simulink model "drive_force_start"  (R2018a)
settings: Solver=ode45  StartTime=0.0  StopTime=15  RelTol=1e-3  EnableMultiTasking=on
PreLoadFcn:
  | load gear_data;
  | FDR = 3.23;
  | AvgEngTorque = 222;
  | Loss = 0.8;
  | r_tire = 1.030;
settings Model: Creator=jrivitus  LastModifiedBy=bneiswan
settings DataIOCC: ExternalInput=[t, gear]  LimitDataPoints=on  LoadExternalInput=on  SaveFormat=Array
settings OptimizationCC: ExpressionDepthLimit=2147483647  LifeSpan=inf
settings DebuggingCC: UnderspecifiedInitializationDetection=Classic  MergeDetectMultiDrivingBlocksExec=none  ParameterPrecisionLossMsg=none  FcnCallInpInsideContextMsg=warning  AllowSymbolicDim=off  StateNameClashWarn=warning  SFUnexpectedBacktrackingDiag=warning  SFNoUnconditionalDefaultTransitionDiag=warning  SFExecutionAtInitializationDiag=none
settings HardwareCC: ProdBitPerPointer=32  ProdBitPerSizeT=32  ProdBitPerPtrDiffT=32  ProdLargestAtomicFloat=None  ProdIntDivRoundTo=Undefined  ProdEndianess=Unspecified  ProdWordSize=32  ProdHWDeviceType=32-bit Generic
settings ModelReferenceCC: PropagateSignalLabelsOutOfModel=off
settings CodeAppCC: StateflowObjectComments=on
settings GRTTargetCC: TargetLangStandard=C89/C90 (ANSI)  GeneratePreprocessorConditionals=Disable all  CombineOutputUpdateFcns=off  GRTInterface=on
settings ConfigComp: CovMetricSettings=dw  CovHtmlReporting=on  CovSaveCumulativeToWorkspaceVar=on  CovSaveSingleToWorkspaceVar=on  CovExternalEMLEnable=off  CovSFcnEnable=off

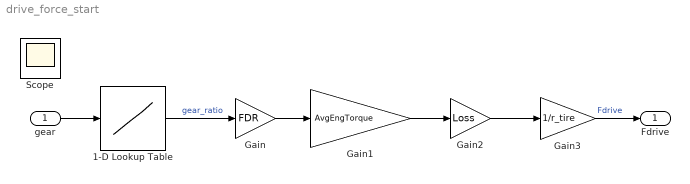
== system drive_force_start ==
  gear : Inport
  1-D Lookup Table : Lookup_n-D  NumberOfTableDimensions=1  BreakpointsForDimension1=[1:5]  Table=[4.21 2.49 1.66 1.24 1.00]  InterpMethod=Flat  ExtrapMethod=Clip  RndMeth=Simplest  InputSameDT=on
  Gain : Gain  Gain=FDR
  Gain1 : Gain  Gain=AvgEngTorque
  Gain2 : Gain  Gain=Loss
  Gain3 : Gain  Gain=1/r_tire
  Fdrive : Outport
  Scope : Scope
  wires:
  gear/1 -> 1-D Lookup Table/1
  1-D Lookup Table/1 -> Gain/1  "gear_ratio"
  Gain/1 -> Gain1/1
  Gain1/1 -> Gain2/1
  Gain2/1 -> Gain3/1
  Gain3/1 -> Fdrive/1  "Fdrive"
